simulink library "asbCubeSatFSWLib"  (R2019a)
settings: Solver=VariableStepAuto  StartTime=0.0  StopTime=10.0  RelTol=1e-3
settings Model: Creator=The MathWorks, Inc.  LastModifiedBy=The MathWorks, Inc.

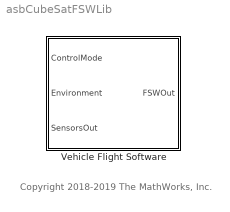
== system asbCubeSatFSWLib ==
  note: Copyright 2018-2019 The MathWorks, Inc.
  Vehicle Flight Software : Subsystem

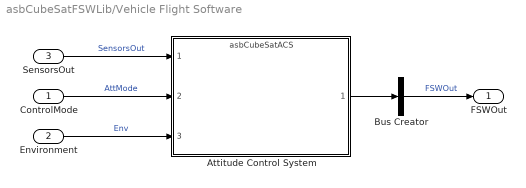
== system asbCubeSatFSWLib/Vehicle Flight Software ==
  ControlMode : Inport
  Environment : Inport  Port=2
  SensorsOut : Inport  Port=3  OutDataTypeStr=Bus: StatesOutBus
  Attitude Control System : ModelReference  ModelNameDialog=asbCubeSatACS.slx  SimulationMode=Normal  ModelReferenceVersion=1.186
  Bus Creator : BusCreator  Inputs=1  OutDataTypeStr=Bus: FCSOutBus  NonVirtualBus=on
  FSWOut : Outport  OutDataTypeStr=Bus: FCSOutBus
  wires:
  Bus Creator/1 -> FSWOut/1  "FSWOut"
  Attitude Control System/1 -> Bus Creator/1
  ControlMode/1 -> Attitude Control System/2  "AttMode"
  SensorsOut/1 -> Attitude Control System/1  "SensorsOut"
  Environment/1 -> Attitude Control System/3  "Env"
